simulink model "hexapod2"  (R2015a)
settings: Solver=ode23tb  StartTime=0.0  StopTime=10  FixedStep=0.0001  MaxStep=0.01  RelTol=1e-4  AbsTol=1e-5
values from neighbouring files (symbols this model uses):
  bH = 1    [runFirst.m]
  C = CM + CL/n^2    (= 0.0001377500155)    [runFirst.m]
  d1 = 0    [runFirst.m]    (also in runFirst2.m)
  d2 = -4.61    [runFirst.m]    (also in runFirst2.m = 0)
  J = JM + JL/n^2    (= 0.008455500031)    [runFirst.m]
  Ka = 12    [runFirst.m]
  Kb = 0.00867    [runFirst.m]
  Ke = 1    [runFirst.m]
  Km = 4.375    [runFirst.m]
  L = 0.0006    [runFirst.m]
  L1 = 3.64    [runFirst.m]    (also in runFirst2.m = 3.4)
  L2 = 5.72    [runFirst.m]    (also in runFirst2.m = 8.7)
  L3 = 12.46    [runFirst.m]    (also in runFirst2.m = 12.73)
  n = 254    [runFirst.m]
  R = 1.4    [runFirst.m]
undefined symbols (not defined in the file or in its folder): bLb, bLs, X, Y, Z
libraries: sm_lib x108, nesl_utility x43, simulink x24, Contact_Forces_Lib x7, roblocks x2
(part 5 of 5)

== system hexapod2/Hexapod/Leg5/Servo/Двигатель ==
  note: ThetaL
  note: OmegaL
  note: OmegaM
  note: TauM
  note: Ia
  note: Vb (противо-ЭДС)
  note: Va-Vb
  note: Va
  note: Vref
  Заданный угол : Inport
  Derivative : Derivative
  Encoder : Gain  Gain=Kb
  Gain : Gain  Gain=Ka
  Gain1 : Gain  Gain=Km
  Gain2 : Gain  Gain=1/n
  Integrator : Integrator
  RL-схема : TransferFcn  Denominator=[L R]
  Saturation3 : Saturate  UpperLimit=90*pi/180  LowerLimit=-90*pi/180  OutMin=[-150*pi/180]  OutMax=[150*pi/180]
  Scope{2..5} (4 alike) : Scope
      Scope3 settings: SaveName=ScopeData4
      Scope4 settings: SaveName=ScopeData5
      Scope5 settings: SaveName=ScopeData6
  Sum : Sum  Inputs=|+-
  Динамика двигателя : TransferFcn  Denominator=[J C]
  Угол : Outport
  Скорость : Outport  Port=2
  Ускорение : Outport  Port=3
  wires:
  RL-схема/1 -> Scope4/1, Gain1/1
  Sum/1 -> RL-схема/1
  Gain1/1 -> Динамика двигателя/1, Scope2/1
  Encoder/1 -> Sum/2
  Динамика двигателя/1 -> Gain2/1, Encoder/1
  Integrator/1 -> Saturation3/1
  Заданный угол/1 -> Gain/1
  Gain2/1 -> Derivative/1, Скорость/1, Integrator/1, Scope3/1
  Gain/1 -> Scope5/1, Sum/1
  Saturation3/1 -> Угол/1
  Derivative/1 -> Ускорение/1

== system hexapod2/Hexapod/Leg5/Servo1/PID ==
  In1 : Inport
  Derivative : Derivative
  Integrator : Integrator
  Kp : Gain  Gain=64
  Kp1 : Gain  Gain=3.4
  Kp2 : Gain  Gain=0
  Sum : Sum  Inputs=|+++
  Out1 : Outport
  wires:
  Derivative/1 -> Sum/3
  Kp/1 -> Sum/2
  Integrator/1 -> Sum/1
  Kp2/1 -> Integrator/1
  Sum/1 -> Out1/1
  Kp1/1 -> Derivative/1
  In1/1 -> Kp/1, Kp1/1, Kp2/1

== system hexapod2/Hexapod/Leg5/Servo1/Двигатель ==
  note: Vref
  note: Va
  note: Va-Vb
  note: Vb (противо-ЭДС)
  note: Ia
  note: TauM
  note: OmegaM
  note: OmegaL
  note: ThetaL
  Заданный угол : Inport
  Derivative : Derivative
  Encoder : Gain  Gain=Kb
  Gain : Gain  Gain=Ka
  Gain1 : Gain  Gain=Km
  Gain2 : Gain  Gain=1/n
  Integrator : Integrator
  RL-схема : TransferFcn  Denominator=[L R]
  Saturation3 : Saturate  UpperLimit=90*pi/180  LowerLimit=-90*pi/180  OutMin=[-150*pi/180]  OutMax=[150*pi/180]
  Scope{2..5} (4 alike) : Scope
      Scope3 settings: SaveName=ScopeData4
      Scope4 settings: SaveName=ScopeData5
      Scope5 settings: SaveName=ScopeData6
  Sum : Sum  Inputs=|+-
  Динамика двигателя : TransferFcn  Denominator=[J C]
  Угол : Outport
  Скорость : Outport  Port=2
  Ускорение : Outport  Port=3
  wires:
  Derivative/1 -> Ускорение/1
  Saturation3/1 -> Угол/1
  Gain/1 -> Sum/1, Scope5/1
  Gain2/1 -> Scope3/1, Integrator/1, Скорость/1, Derivative/1
  Заданный угол/1 -> Gain/1
  Integrator/1 -> Saturation3/1
  Динамика двигателя/1 -> Encoder/1, Gain2/1
  Encoder/1 -> Sum/2
  Gain1/1 -> Scope2/1, Динамика двигателя/1
  Sum/1 -> RL-схема/1
  RL-схема/1 -> Gain1/1, Scope4/1

== system hexapod2/Hexapod/Leg5/Servo2/PID ==
  In1 : Inport
  Derivative : Derivative
  Integrator : Integrator
  Kp : Gain  Gain=64
  Kp1 : Gain  Gain=3.4
  Kp2 : Gain  Gain=0
  Sum : Sum  Inputs=|+++
  Out1 : Outport
  wires:
  In1/1 -> Kp2/1, Kp1/1, Kp/1
  Kp1/1 -> Derivative/1
  Sum/1 -> Out1/1
  Kp2/1 -> Integrator/1
  Integrator/1 -> Sum/1
  Kp/1 -> Sum/2
  Derivative/1 -> Sum/3

== system hexapod2/Hexapod/Leg5/Servo2/Двигатель ==
  note: ThetaL
  note: OmegaL
  note: OmegaM
  note: TauM
  note: Ia
  note: Vb (противо-ЭДС)
  note: Va-Vb
  note: Va
  note: Vref
  Заданный угол : Inport
  Derivative : Derivative
  Encoder : Gain  Gain=Kb
  Gain : Gain  Gain=Ka
  Gain1 : Gain  Gain=Km
  Gain2 : Gain  Gain=1/n
  Integrator : Integrator
  RL-схема : TransferFcn  Denominator=[L R]
  Saturation3 : Saturate  UpperLimit=90*pi/180  LowerLimit=-90*pi/180  OutMin=[-150*pi/180]  OutMax=[150*pi/180]
  Scope{2..5} (4 alike) : Scope
      Scope3 settings: SaveName=ScopeData4
      Scope4 settings: SaveName=ScopeData5
      Scope5 settings: SaveName=ScopeData6
  Sum : Sum  Inputs=|+-
  Динамика двигателя : TransferFcn  Denominator=[J C]
  Угол : Outport
  Скорость : Outport  Port=2
  Ускорение : Outport  Port=3
  wires:
  RL-схема/1 -> Scope4/1, Gain1/1
  Sum/1 -> RL-схема/1
  Gain1/1 -> Динамика двигателя/1, Scope2/1
  Encoder/1 -> Sum/2
  Динамика двигателя/1 -> Gain2/1, Encoder/1
  Integrator/1 -> Saturation3/1
  Заданный угол/1 -> Gain/1
  Gain2/1 -> Derivative/1, Скорость/1, Integrator/1, Scope3/1
  Gain/1 -> Scope5/1, Sum/1
  Saturation3/1 -> Угол/1
  Derivative/1 -> Ускорение/1

== system hexapod2/Hexapod/Leg6/Servo/PID ==
  In1 : Inport
  Derivative : Derivative
  Integrator : Integrator
  Kp : Gain  Gain=64
  Kp1 : Gain  Gain=3.4
  Kp2 : Gain  Gain=0
  Sum : Sum  Inputs=|+++
  Out1 : Outport
  wires:
  Derivative/1 -> Sum/3
  Kp/1 -> Sum/2
  Integrator/1 -> Sum/1
  Kp2/1 -> Integrator/1
  Sum/1 -> Out1/1
  Kp1/1 -> Derivative/1
  In1/1 -> Kp/1, Kp1/1, Kp2/1

== system hexapod2/Hexapod/Leg6/Servo/Двигатель ==
  note: Vref
  note: Va
  note: Va-Vb
  note: Vb (противо-ЭДС)
  note: Ia
  note: TauM
  note: OmegaM
  note: OmegaL
  note: ThetaL
  Заданный угол : Inport
  Derivative : Derivative
  Encoder : Gain  Gain=Kb
  Gain : Gain  Gain=Ka
  Gain1 : Gain  Gain=Km
  Gain2 : Gain  Gain=1/n
  Integrator : Integrator
  RL-схема : TransferFcn  Denominator=[L R]
  Saturation3 : Saturate  UpperLimit=90*pi/180  LowerLimit=-90*pi/180  OutMin=[-150*pi/180]  OutMax=[150*pi/180]
  Scope{2..5} (4 alike) : Scope
      Scope3 settings: SaveName=ScopeData4
      Scope4 settings: SaveName=ScopeData5
      Scope5 settings: SaveName=ScopeData6
  Sum : Sum  Inputs=|+-
  Динамика двигателя : TransferFcn  Denominator=[J C]
  Угол : Outport
  Скорость : Outport  Port=2
  Ускорение : Outport  Port=3
  wires:
  Derivative/1 -> Ускорение/1
  Saturation3/1 -> Угол/1
  Gain/1 -> Sum/1, Scope5/1
  Gain2/1 -> Scope3/1, Integrator/1, Скорость/1, Derivative/1
  Заданный угол/1 -> Gain/1
  Integrator/1 -> Saturation3/1
  Динамика двигателя/1 -> Encoder/1, Gain2/1
  Encoder/1 -> Sum/2
  Gain1/1 -> Scope2/1, Динамика двигателя/1
  Sum/1 -> RL-схема/1
  RL-схема/1 -> Gain1/1, Scope4/1

== system hexapod2/Hexapod/Leg6/Servo1/PID ==
  In1 : Inport
  Derivative : Derivative
  Integrator : Integrator
  Kp : Gain  Gain=64
  Kp1 : Gain  Gain=3.4
  Kp2 : Gain  Gain=0
  Sum : Sum  Inputs=|+++
  Out1 : Outport
  wires:
  In1/1 -> Kp2/1, Kp1/1, Kp/1
  Kp1/1 -> Derivative/1
  Sum/1 -> Out1/1
  Kp2/1 -> Integrator/1
  Integrator/1 -> Sum/1
  Kp/1 -> Sum/2
  Derivative/1 -> Sum/3

== system hexapod2/Hexapod/Leg6/Servo1/Двигатель ==
  note: ThetaL
  note: OmegaL
  note: OmegaM
  note: TauM
  note: Ia
  note: Vb (противо-ЭДС)
  note: Va-Vb
  note: Va
  note: Vref
  Заданный угол : Inport
  Derivative : Derivative
  Encoder : Gain  Gain=Kb
  Gain : Gain  Gain=Ka
  Gain1 : Gain  Gain=Km
  Gain2 : Gain  Gain=1/n
  Integrator : Integrator
  RL-схема : TransferFcn  Denominator=[L R]
  Saturation3 : Saturate  UpperLimit=90*pi/180  LowerLimit=-90*pi/180  OutMin=[-150*pi/180]  OutMax=[150*pi/180]
  Scope{2..5} (4 alike) : Scope
      Scope3 settings: SaveName=ScopeData4
      Scope4 settings: SaveName=ScopeData5
      Scope5 settings: SaveName=ScopeData6
  Sum : Sum  Inputs=|+-
  Динамика двигателя : TransferFcn  Denominator=[J C]
  Угол : Outport
  Скорость : Outport  Port=2
  Ускорение : Outport  Port=3
  wires:
  RL-схема/1 -> Scope4/1, Gain1/1
  Sum/1 -> RL-схема/1
  Gain1/1 -> Динамика двигателя/1, Scope2/1
  Encoder/1 -> Sum/2
  Динамика двигателя/1 -> Gain2/1, Encoder/1
  Integrator/1 -> Saturation3/1
  Заданный угол/1 -> Gain/1
  Gain2/1 -> Derivative/1, Скорость/1, Integrator/1, Scope3/1
  Gain/1 -> Scope5/1, Sum/1
  Saturation3/1 -> Угол/1
  Derivative/1 -> Ускорение/1

== system hexapod2/Hexapod/Leg6/Servo2/PID ==
  In1 : Inport
  Derivative : Derivative
  Integrator : Integrator
  Kp : Gain  Gain=64
  Kp1 : Gain  Gain=3.4
  Kp2 : Gain  Gain=0
  Sum : Sum  Inputs=|+++
  Out1 : Outport
  wires:
  Derivative/1 -> Sum/3
  Kp/1 -> Sum/2
  Integrator/1 -> Sum/1
  Kp2/1 -> Integrator/1
  Sum/1 -> Out1/1
  Kp1/1 -> Derivative/1
  In1/1 -> Kp/1, Kp1/1, Kp2/1

== system hexapod2/Hexapod/Leg6/Servo2/Двигатель ==
  note: Vref
  note: Va
  note: Va-Vb
  note: Vb (противо-ЭДС)
  note: Ia
  note: TauM
  note: OmegaM
  note: OmegaL
  note: ThetaL
  Заданный угол : Inport
  Derivative : Derivative
  Encoder : Gain  Gain=Kb
  Gain : Gain  Gain=Ka
  Gain1 : Gain  Gain=Km
  Gain2 : Gain  Gain=1/n
  Integrator : Integrator
  RL-схема : TransferFcn  Denominator=[L R]
  Saturation3 : Saturate  UpperLimit=90*pi/180  LowerLimit=-90*pi/180  OutMin=[-150*pi/180]  OutMax=[150*pi/180]
  Scope{2..5} (4 alike) : Scope
      Scope3 settings: SaveName=ScopeData4
      Scope4 settings: SaveName=ScopeData5
      Scope5 settings: SaveName=ScopeData6
  Sum : Sum  Inputs=|+-
  Динамика двигателя : TransferFcn  Denominator=[J C]
  Угол : Outport
  Скорость : Outport  Port=2
  Ускорение : Outport  Port=3
  wires:
  Derivative/1 -> Ускорение/1
  Saturation3/1 -> Угол/1
  Gain/1 -> Sum/1, Scope5/1
  Gain2/1 -> Scope3/1, Integrator/1, Скорость/1, Derivative/1
  Заданный угол/1 -> Gain/1
  Integrator/1 -> Saturation3/1
  Динамика двигателя/1 -> Encoder/1, Gain2/1
  Encoder/1 -> Sum/2
  Gain1/1 -> Scope2/1, Динамика двигателя/1
  Sum/1 -> RL-схема/1
  RL-схема/1 -> Gain1/1, Scope4/1
